simulink model "sensor_test"  (R2022b)
settings: Solver=FixedStepDiscrete  StartTime=0.0  StopTime=10.0  RelTol=1e-3
InitFcn:
  | mbd_s32k_consistency_checks(bdroot(gcs));
undefined symbols (not defined in the file or in its folder): LQFP
libraries: mbd_s32k1xx_ec_toolbox x10
settings Model: Creator=termi  LastModifiedBy=termi
settings DataIOCC: ExternalInput=off  InitialState=off  SaveOutput=off  SignalLogging=off  SaveTime=off
settings OptimizationCC: DefaultParameterBehavior=Inlined  EnhancedBackFolding=on  PassReuseOutputArgsAs=Individual arguments  ZeroExternalMemoryAtStartup=off  ZeroInternalMemoryAtStartup=off  OptimizeBlockOrder=speed  DifferentSizesBufferReuse=on  OptimizationCustomize=off  EfficientTunableParamExpr=on
settings DebuggingCC: InheritedTsInSrcMsg=none  SingleTaskRateTransMsg=error  ParameterTunabilityLossMsg=error  UnconnectedInputMsg=error  UnconnectedOutputMsg=error  UnconnectedLineMsg=error  UnknownTsInhSupMsg=error
settings HardwareCC: ProdBitPerPointer=32  ProdBitPerSizeT=32  ProdBitPerPtrDiffT=32  ProdLargestAtomicInteger=Long  ProdLargestAtomicFloat=Double  ProdWordSize=32  ProdHWDeviceType=ARM Compatible->ARM Cortex
settings SFSimCC: MATLABDynamicMemAlloc=off
settings RTWCC: Description=Model Based Design Toolbox S32K1xx Code Generation Target  SystemTargetFile=mbd_s32k.tlc  MakeCommand=mbd_s32k_make_rtw COPY_MDLREF_INCLUDES=0  TemplateMakefile=mbd_s32k.tmf
settings CodeAppCC: ForceParamTrailComments=on  IgnoreCustomStorageClasses=off  OperatorAnnotations=on  SimulinkDataObjDesc=on  SFDataObjDesc=on  InsertBlockDesc=on
settings STFCustomTargetCC: TargetLangStandard=C99 (ISO)  MultiwordLength=256  GenerateSampleERTMain=on  CombineOutputUpdateFcns=on  ERTCustomFileBanners=on  SupportContinuousTime=off  SupportNonInlinedSFcns=off  RemoveResetFunc=on  MATLABClassNameForMDSCustomization=Simulink.SoftwareTarget.ERTCustomization  SystemTargetFile=mbd_s32k.tlc
settings ERTTargetCC: TargetLangStandard=C99 (ISO)  GenerateSampleERTMain=on  ParMdlRefBuildCompliant=off  CompOptLevelCompliant=off  ConcurrentExecutionCompliant=off  ModelStepFunctionPrototypeControlCompliant=off  CPPClassGenCompliant=off  UseToolchainInfoCompliant=off  InlinedParameterPlacement=NonHierarchical  ERTSrcFileBannerTemplate=mbd_ert_code_template.cgt  ERTHdrFileBannerTemplate=mbd_ert_code_template.cgt  ERTDataSrcFileTemplate=mbd_ert_code_template.cgt  ERTDataHdrFileTemplate=mbd_ert_code_template.cgt  ERTCustomFileTemplate=example_file_process.tlc

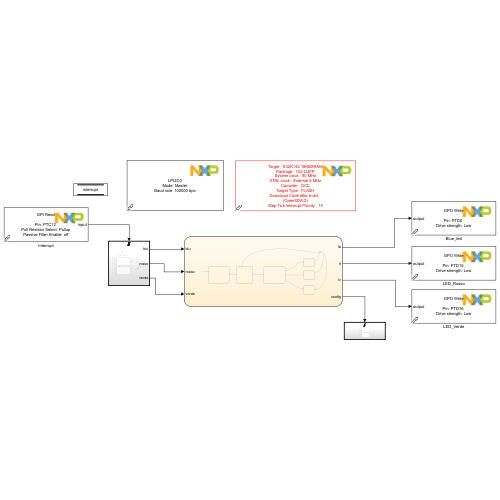
[thumbnail: Simulink's stored preview of the top-level diagram]
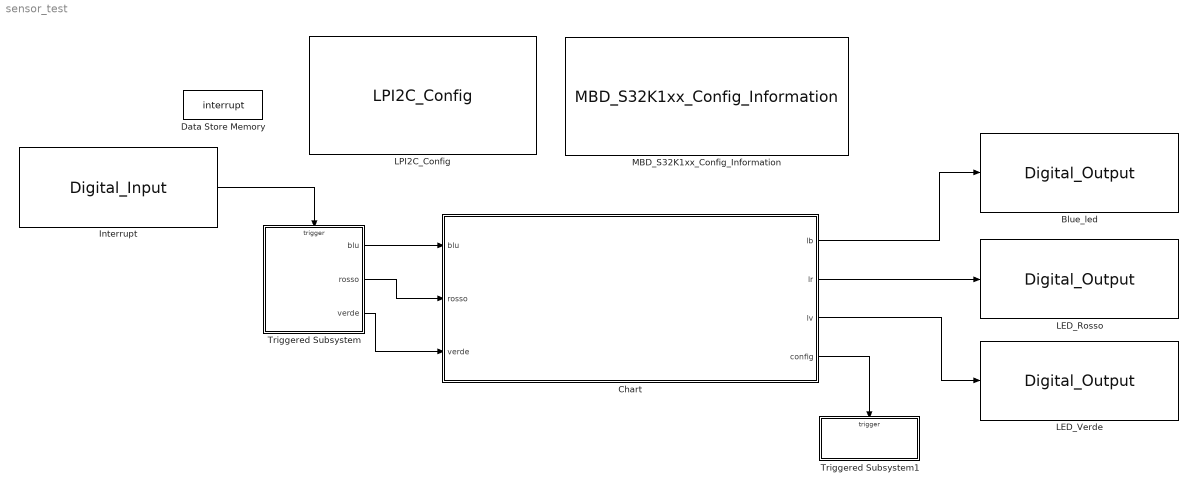
== system sensor_test ==
  Blue_led : mbd_s32k1xx_ec_toolbox/GPIO Blocks/Digital_Output  gpio_pin=PTD0: [PTD0 | Port D I/O]  init_val=Low  drive_strength=Low
  Chart : Stateflow chart  TreatAsAtomicUnit=on
  Data Store Memory : DataStoreMemory  DataStoreName=interrupt  WriteAfterWriteMsg=warning  ShowAdditionalParam=off
  Interrupt : mbd_s32k1xx_ec_toolbox/GPIO Blocks/Digital_Input  gpio_pin=PTC12: [PTC12 | Port C I/O]  pull_resistor=Pullup  passive_filter=off
  LED_Rosso : mbd_s32k1xx_ec_toolbox/GPIO Blocks/Digital_Output  gpio_pin=PTD15: [PTD15 | Port D I/O]  init_val=Low  drive_strength=Low
  LED_Verde : mbd_s32k1xx_ec_toolbox/GPIO Blocks/Digital_Output  gpio_pin=PTD16: [PTD16 | Port D I/O]  init_val=Low  drive_strength=Low
  LPI2C_Config : mbd_s32k1xx_ec_toolbox/Communication Blocks/I2C Blocks/LPI2C_Config  instance=0  mode=Master  opmode=Standard (up to 100 kbit/s)  bdr=100000  addr=1  is10bitaddr=off  status=off  sda=PTA2: [LPI2C0_SDA | LPI2C Data I/O]  scl=PTA3: [LPI2C0_SCL | LPI2C Clock I/O]
  MBD_S32K1xx_Config_Information : mbd_s32k1xx_ec_toolbox/MBD_S32K1xx_Config_Information  Priority=1  mbdt_ver=0  disp_str=|  config_params=[]  mcu_target_name=S32K142  mcu_target_package=100-LQFP  mcu_target_sram_size=16KB  mcu_system_clock_freq=80  mcu_xtal_freq=External 8  mcu_steptick_timer=LPIT Channel 0  mcu_steptick_prio=15  ds_import_enable=on  target_compiler=GCC  target_memory=FLASH  gcc_target_compile_opts=-mthumb -mfloat-abi=hard -mfpu=fpv4-sp-d16 -O1 -g -gstrict-dwarf  gcc_target_assemble_opts=-mthumb -mfloat-abi=hard -mfpu=fpv4-sp-d16 -g  gcc_target_link_opts=-mthumb -mfloat-abi=hard -mfpu=fpv4-sp-d16  gcc_target_default_lcf=on  gcc_target_user_lcf=S32K142_16_flash.ld  ghs_target_compile_opts=-cpu=cortexm4f -thumb -fpu=vfpv4_d16 -fsingle -Ogeneral -Wundef -Wimplicit-int -Wshadow -Wtrigraphs --no_commons --gnu_asm -gnu99 -gdwarf-2 -G  ghs_target_assemble_opts=-cpu=cortexm4f -fpu=vfpv4_d16  ghs_target_link_opts=-cpu=cortexm4f -thumb -fpu=vfpv4_d16  ghs_target_default_lcf=on  ghs_target_user_lcf=S32K142_16_flash.ld  iar_target_compile_opts=--cpu=Cortex-M4F --thumb --fpu=VFPv4_sp -Ol -e --debug --dlib_config normal  iar_target_assemble_opts=--cpu Cortex-M4F --thumb --fpu VFPv4_sp  iar_target_link_opts=--no_exceptions --vfe --inline  iar_target_default_lcf=on  iar_target_user_lcf=S32K142_16_flash.icf  pil_download_enable=off  rbl_download_enable=on  rbl_start_delay=5000  rbl_download_interface=OpenSDA  rbl_restart_request=off  rbl_com_port=Custom  rbl_com_port_custom=COM3  pil_download_rate=115200  pil_download_rate_custom=115200  pil_opensda_drive=Custom  pil_opensda_drive_custom=D  jtag_interface=OpenSDA Embedded Debug  jlink_default_path=on  jlink_user_path=C:\Program Files\SEGGER\JLink\  pil_uart_instance=1  pil_uart_rx=PTC6: [LPUART1_RX | Receive]  pil_uart_tx=PTC7: [LPUART1_TX | Transmit]  FTM_PWM_PcrCheckEnDis=on  FTM_Input_Edge_Inputs_PcrCheckEnDis=on  FTM_Dual_Edge_Inputs_PcrCheckEnDis=on  FTM_Quadrature_Inputs_PcrCheckEnDis=on  FTM_Hall_Sensor_Inputs_PcrCheckEnDis=on  LPTMR_PcrCheckEnDis=on  PIT_PcrCheckEnDis=on  RTC_PcrCheckEnDis=on  FlexCAN_PcrCheckEnDis=on  LIN_PcrCheckEnDis=on  FlexIO_PcrCheckEnDis=on  LPI2C_PcrCheckEnDis=on  LPSPI_PcrCheckEnDis=on  LPUART_PcrCheckEnDis=on  CMP_PcrCheckEnDis=on  GPIO_OutputPcrCheckEnDis=on  GPIO_InputPcrCheckEnDis=on  SBC_PcrCheckEnDis=on  BMS_PcrCheckEnDis=on  AMMCLIB_PcrCheckEnDis=on  FM_PcrCheckEnDis=on  Profile_PcrCheckEnDis=on  ConfigParams_PcrCheckEnDis=on  ModelRef_PcrCheckEnDis=on  PDB0_PcrCheckEnDis=on  CSEc_PcrCheckEnDis=on  eDMA_PcrCheckEnDis=on  FLASH_PcrCheckEnDis=on  ADC_PcrCheckEnDis=on  WDOG_PcrCheckEnDis=on
      | Target : S32K144-64KB_SRAM
      | Package : 100-pin
      | System clock : 80 MHz
      | XTAL clock : External 8 MHz
      | Compiler : IAR
      | Target Type : FLASH
      | Download Code after build : off
      | Step Tick Interrupt Priority : 15
  Triggered Subsystem : Subsystem  TreatAsAtomicUnit=on
  Triggered Subsystem1 : Subsystem  TreatAsAtomicUnit=on
  wires:
  Chart/2(lr) -> LED_Rosso/1
  Chart/3(lv) -> LED_Verde/1
  Chart/1(lb) -> Blue_led/1
  Interrupt/1 -> Triggered Subsystem/Trigger
  Chart/4(config) -> Triggered Subsystem1/Trigger
  Triggered Subsystem/1(blu) -> Chart/1(blu)
  Triggered Subsystem/2(rosso) -> Chart/2(rosso)
  Triggered Subsystem/3(verde) -> Chart/3(verde)

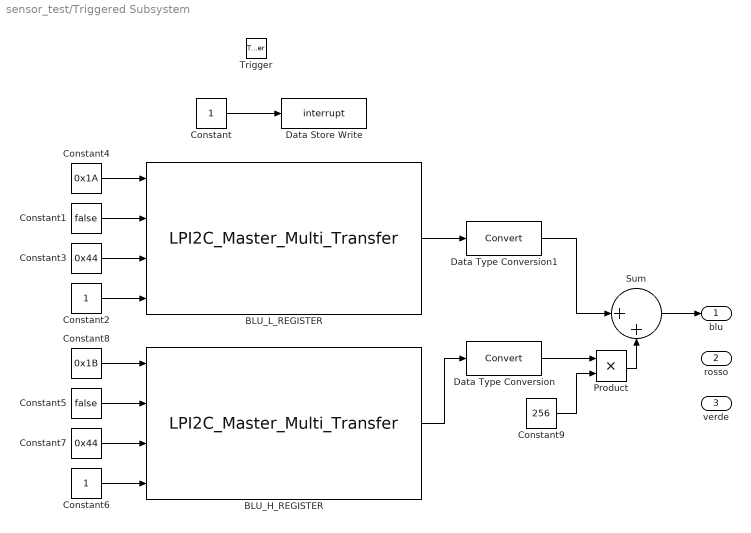
== system sensor_test/Triggered Subsystem ==
  Trigger : TriggerPort  VariantControl=(inherit)
  BLU_H_REGISTER : mbd_s32k1xx_ec_toolbox/Communication Blocks/I2C Blocks/LPI2C_Master_Multi_Transfer  instance=0  xfermode=Blocking  Timeout=28.8  delay_between_transfers=28.8  is10bit=off  status=off
  BLU_L_REGISTER : mbd_s32k1xx_ec_toolbox/Communication Blocks/I2C Blocks/LPI2C_Master_Multi_Transfer  instance=0  xfermode=Blocking  Timeout=28.8  delay_between_transfers=28.8  is10bit=off  status=off
  Constant : Constant
  Constant1 : Constant  Value=false
  Constant2 : Constant
  Constant3 : Constant  Value=0x44
  Constant4 : Constant  Value=0x1A
  Constant5 : Constant  Value=false
  Constant6 : Constant
  Constant7 : Constant  Value=0x44
  Constant8 : Constant  Value=0x1B
  Constant9 : Constant  Value=256
  Data Store Write : DataStoreWrite  DataStoreName=interrupt  IndexOptions=Index vector (dialog)  Indices=1  OutputSizes=1
  Data Type Conversion : DataTypeConversion  SaturateOnIntegerOverflow=off  RndMeth=Floor
  Data Type Conversion1 : DataTypeConversion  SaturateOnIntegerOverflow=off  RndMeth=Floor
  Product : Product
  Sum : Sum  Inputs=|++
  blu : Outport
  rosso : Outport  Port=2
  verde : Outport  Port=3
  wires:
  Constant/1 -> Data Store Write/1
  Constant3/1 -> BLU_L_REGISTER/3
  Constant2/1 -> BLU_L_REGISTER/4
  Constant1/1 -> BLU_L_REGISTER/2
  Constant4/1 -> BLU_L_REGISTER/1
  Constant6/1 -> BLU_H_REGISTER/4
  Constant5/1 -> BLU_H_REGISTER/2
  Constant7/1 -> BLU_H_REGISTER/3
  Constant8/1 -> BLU_H_REGISTER/1
  Product/1 -> Sum/2
  Constant9/1 -> Product/2
  Sum/1 -> blu/1
  Data Type Conversion/1 -> Product/1
  BLU_H_REGISTER/1 -> Data Type Conversion/1
  BLU_L_REGISTER/1 -> Data Type Conversion1/1
  Data Type Conversion1/1 -> Sum/1

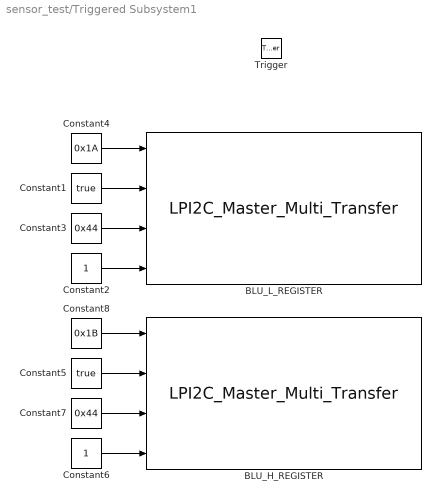
== system sensor_test/Triggered Subsystem1 ==
  Trigger : TriggerPort  VariantControl=(inherit)
  BLU_H_REGISTER : mbd_s32k1xx_ec_toolbox/Communication Blocks/I2C Blocks/LPI2C_Master_Multi_Transfer  instance=0  xfermode=Blocking  Timeout=28.8  delay_between_transfers=28.8  is10bit=off  status=off
  BLU_L_REGISTER : mbd_s32k1xx_ec_toolbox/Communication Blocks/I2C Blocks/LPI2C_Master_Multi_Transfer  instance=0  xfermode=Blocking  Timeout=28.8  delay_between_transfers=28.8  is10bit=off  status=off
  Constant1 : Constant  Value=true
  Constant2 : Constant
  Constant3 : Constant  Value=0x44
  Constant4 : Constant  Value=0x1A
  Constant5 : Constant  Value=true
  Constant6 : Constant
  Constant7 : Constant  Value=0x44
  Constant8 : Constant  Value=0x1B
  wires:
  Constant3/1 -> BLU_L_REGISTER/3
  Constant2/1 -> BLU_L_REGISTER/4
  Constant1/1 -> BLU_L_REGISTER/2
  Constant4/1 -> BLU_L_REGISTER/1
  Constant6/1 -> BLU_H_REGISTER/4
  Constant5/1 -> BLU_H_REGISTER/2
  Constant7/1 -> BLU_H_REGISTER/3
  Constant8/1 -> BLU_H_REGISTER/1

== stateflow chart sensor_test/Chart ==
  note: sensing == 1 -> BLU
      | sensing == 2 -> ROSSO
      | sensing == 3 -> VERDE
  state blu_On
    en:
    lb  = 1;
  state Sensor_init
    en:
    config = 1;
    h_th = 300;
    l_th = 10;
  state wait
    en:
    lb = 0;
    lr = 0;
    lr = 0;
    interrupt = 0;
  state Color_detection
    en:
    switch true
    case blu > h_th
    sensing = 1;
    case rosso > h_th
    sensing = 2;
    case verde > h_th
    sensing = 3
    end
  state rosso_on
    en:
    lr  = 1;
  state verde_on
    en:
    lv  = 1;
  (junction 15) -> wait : [after (10,sec)]
  verde_on -> (junction 15)
  rosso_on -> (junction 15)
  blu_On -> (junction 15)
  Color_detection -> blu_On [order 1] : [sensing == 1]
  (default) -> Sensor_init
  wait -> Color_detection : [interrupt == 1]
  Sensor_init -> wait
  Color_detection -> rosso_on [order 2] : [sensing == 2]
  Color_detection -> verde_on [order 3] : [sensing == 3]
  data: lb output; lr output; lv output; interrupt data_store_memory; blu input; rosso input; verde input; h_th local; l_th local; config output; sensing local
